simulink model "tank_Pm_solved"  (R2025b)
settings: Solver=VariableStepAuto  StartTime=0.0  StopTime=10.0  RelTol=1e-3
model workspace (MAT data in the model file):
  P0 = Simulink.Parameter
  P0.Value = 300
  P0.Complexity = 'real'
  P0.Dimensions = [1 1]
  P0.DataType = 'auto'
  T0 = Simulink.Parameter
  T0.Value = 40.5939137189
  T0.Complexity = 'real'
  T0.Dimensions = [1 1]
  T0.DataType = 'auto'
  mdotGain = Simulink.Parameter
  mdotGain.Value = 1.59005652853e-08
  mdotGain.Complexity = 'real'
  mdotGain.Dimensions = [1 1]
  mdotGain.DataType = 'auto'
undefined symbols (not defined in the file): gamma, Patm, R, ts, V
settings Model: Creator=karadeli  LastModifiedBy=karadeli

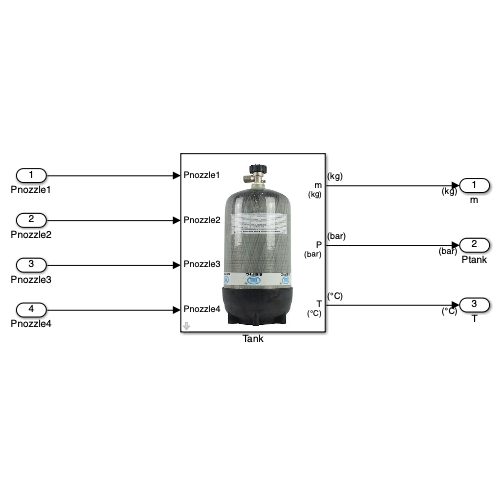
[thumbnail: Simulink's stored preview of the top-level diagram]
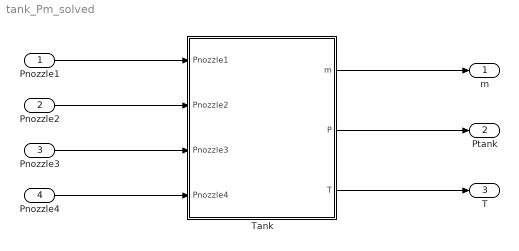
== system tank_Pm_solved ==
  Pnozzle1 : Inport
  Pnozzle2 : Inport  Port=2
  Pnozzle3 : Inport  Port=3
  Pnozzle4 : Inport  Port=4
  Tank : Subsystem  mask{P0=300, T0=40.5939, mdotGain=1.5900565285340063E-8}
      mask Display: image('Tank.png');
  m : Outport  Unit=kg
  Ptank : Outport  Port=2  Unit=bar
  T : Outport  Port=3  Unit=°C
  wires:
  Pnozzle1/1 -> Tank/1(Pnozzle1)
  Tank/1(m) -> m/1
  Tank/2(P) -> Ptank/1
  Pnozzle2/1 -> Tank/2(Pnozzle2)
  Pnozzle3/1 -> Tank/3(Pnozzle3)
  Pnozzle4/1 -> Tank/4(Pnozzle4)
  Tank/3(T) -> T/1

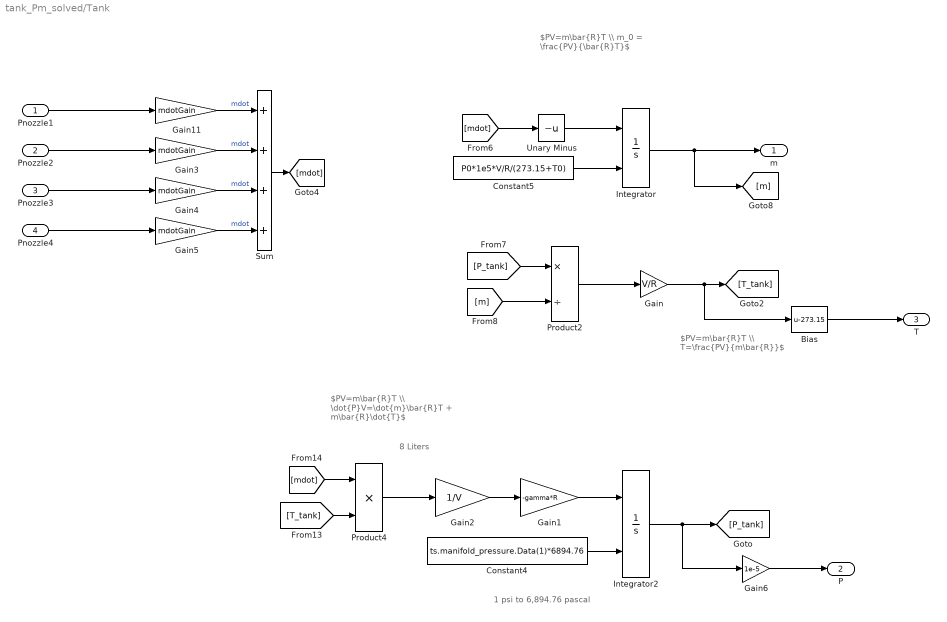
== system tank_Pm_solved/Tank ==
  note: 8 Liters
  note: $PV=m\bar{R}T \\ T=\frac{PV}{m\bar{R}}$
  note: 1 psi to 6,894.76 pascal
  note: $PV=m\bar{R}T \\ \dot{P}V=\dot{m}\bar{R}T + m\bar{R}\dot{T}$
  note: $PV=m\bar{R}T \\ m_0 = \frac{PV}{\bar{R}T}$
  Pnozzle1 : Inport
  Pnozzle2 : Inport  Port=2
  Pnozzle3 : Inport  Port=3
  Pnozzle4 : Inport  Port=4
  Bias : Bias  Bias=-273.15  SaturateOnIntegerOverflow=off
  Constant4 : Constant  Value=ts.manifold_pressure.Data(1)*6894.76
  Constant5 : Constant  Value=P0*1e5*V/R/(273.15+T0)
  Gain : Gain  Gain=V/R
  Gain1 : Gain  Gain=-gamma*R
  Gain{3..5,11} (4 alike) : Gain  Gain=mdotGain
  Gain2 : Gain  Gain=1/V
  Gain6 : Gain  Gain=1e-5
  Integrator : Integrator  InitialConditionSource=external  InitialCondition=3  LimitOutput=on  UpperSaturationLimit=5  LowerSaturationLimit=Patm*V/R/100
  Integrator2 : Integrator  InitialConditionSource=external  InitialCondition=16719786.44
  Product2 : Product  Inputs=*/
  Product4 : Product
  Sum : Sum  Inputs=4
  Unary Minus : UnaryMinus
  m : Outport  Unit=kg
  P : Outport  Port=2  Unit=bar
  T : Outport  Port=3  Unit=°C
  wires:
  [P_tank] -> Product2/1
  [mdot] -> Product4/1
  Constant4/1 -> Integrator2/2
  Product4/1 -> Gain2/1
  [m] -> Product2/2
  [T_tank] -> Product4/2
  Product2/1 -> Gain/1
  Integrator2/1 -> Gain6/1, [P_tank]
  Gain11/1 -> Sum/1  "mdot"
  Gain/1 -> Bias/1, [T_tank]
  Pnozzle1/1 -> Gain11/1
  Unary Minus/1 -> Integrator/1
  Integrator/1 -> m/1, [m]
  Gain1/1 -> Integrator2/1
  [mdot] -> Unary Minus/1
  Gain2/1 -> Gain1/1
  Constant5/1 -> Integrator/2
  Pnozzle2/1 -> Gain3/1
  Pnozzle3/1 -> Gain4/1
  Pnozzle4/1 -> Gain5/1
  Gain5/1 -> Sum/4  "mdot"
  Gain4/1 -> Sum/3  "mdot"
  Gain3/1 -> Sum/2  "mdot"
  Sum/1 -> [mdot]
  Bias/1 -> T/1
  Gain6/1 -> P/1
